simulink model "VCU10"  (R2021b)
settings: Solver=FixedStepDiscrete  StartTime=0.0  StopTime=10.0  FixedStep=0.01  RelTol=1e-3
values from neighbouring files (symbols this model uses):
  F = 0.0    [VCU10DB.sldd]
  FSEC_ESP_EMERGENCY_PRESSURE_MPA = 8.0    [VCU10DB.sldd]
  T = 1.0    [VCU10DB.sldd]
libraries: simulink x148, hdlsllib x90
(part 4 of 4)

== matlab function VCU10/DBC_Debug_StatusPack ==
  data: status_base input; status output; model_lox input; model_hox input
function status = dbg_status_pack(status_base, model_lox, model_hox)
%#codegen
status = uint8(status_base);
status(5) = uint8(model_lox);
status(6) = uint8(model_hox);
end

== stateflow chart VCU10/TS_Activation/Chart1 ==
  state Ignition_Check
    state begin
      run_flag=0;
    state Run_Check_Flag
      (default) -> (junction 5)
      (junction 5) -> (junction 7) [order 1] : [run_button==0]
      (junction 5) -> (junction 9) [order 2] : {run_check_flag=0;}
      (junction 7) -> (junction 8) : {run_check_flag=1;}
      (junction 8) -> (junction 9)
      (junction 9) -> (junction 10)
    state Check
      (default) -> (junction 23)
      (junction 23) -> (junction 25) [order 1] : [run_button==1]
      (junction 23) -> (junction 29) [order 2]
      (junction 25) -> (junction 27) : {run_flag=1;run=T;}
      (junction 27) -> (junction 29)
      (junction 29) -> (junction 32)
    (default) -> begin
    begin -> Run_Check_Flag
    (junction 17) -> Run_Check_Flag [order 2] : [run_check_flag==0]
    Check -> (junction 17)
    (junction 17) -> Check [order 1] : [run_check_flag==1]
    Run_Check_Flag -> (junction 17)
  state Flameout_Check
    state Run_Offcheck_Flag
      (default) -> (junction 39)
      (junction 39) -> (junction 42) [order 1] : [run_button==0]
      (junction 42) -> (junction 44) : {run_offcheck_flag=1;}
      (junction 39) -> (junction 46) [order 2] : {run_offcheck_flag}
      (junction 44) -> (junction 46)
      (junction 46) -> (junction 49)
    state Checkoff
      (default) -> (junction 63)
      (junction 63) -> (junction 61) [order 1] : [run_button==1]
      (junction 63) -> (junction 57) [order 2]
      (junction 61) -> (junction 60) : {run_flag=0;run=F;}
      (junction 60) -> (junction 57)
      (junction 57) -> (junction 58)
    (default) -> Run_Offcheck_Flag
    (junction 52) -> Run_Offcheck_Flag [order 1] : [run_offcheck_flag==0]
    (junction 52) -> Checkoff [order 3]
    (junction 52) -> Checkoff [order 2] : [run_offcheck_flag==1]
    Run_Offcheck_Flag -> (junction 52)
  (default) -> Ignition_Check
  Ignition_Check -> Flameout_Check : [run_flag==1]
  Flameout_Check -> Ignition_Check : [run_flag==0]
  data: run_button input; run output boolean; run_check_flag local =0; run_offcheck_flag local =0; run_flag local =0; T parameter; F parameter

== stateflow chart VCU10/TS_Activation/Chart2 ==
  state begin
  state delay
  (default) -> begin
  begin -> (junction 5) : {ts=0}
  (junction 5) -> (junction 11) : [tsms_button==1]
  (junction 11) -> (junction 35) : [di8==1]
  (junction 35) -> (junction 36) [order 2] : [as_flag==1]
  (junction 35) -> (junction 7) [order 1] : [as_flag==0]
  (junction 7) -> delay : [run==1&&brake_on==1]{ts=1;ts_warning=T}
  (junction 36) -> delay : {ts=1}
  delay -> (junction 30) : after(2,sec)
  (junction 30) -> (junction 9) : {ts_warning=F}
  (junction 9) -> (junction 13) : [tsms_button==0||di8==0||run==0]{ts=0}
  (junction 13) -> (junction 15)
  data: ts output; di8 input; run input; tsms_button input; brake_on input; ts_warning output; T parameter; F parameter; as_flag input

== stateflow chart VCU10/Res/Res_Msg/Subsystem/heaartbeat_chart ==
  state begin
  state compare
    res_hbcheck=1;
  state same
    hbcnt = hbcnt + 1;
  state judge
    res_hbcheck=0;
  (default) -> begin
  begin -> compare : [hasChanged(res_heartbeat)]
  judge -> compare : [hasChanged(res_heartbeat)]{hbcnt=0}
  same -> compare [order 2] : [hasChanged(res_heartbeat)]{hbcnt=0}
  compare -> same : [~hasChanged(res_heartbeat)]
  same -> judge [order 1] : [hbcnt>30]
  data: res_heartbeat input; res_hbcheck output; hbcnt local

== stateflow chart VCU10/Buzzer/Chart ==
  state Default
    en:
    ebs_buzzer=F;
  state Emergency
    en:
    ebs_buzzer=T;
  (default) -> Default
  Default -> Emergency : [as_emergency_flag==1]
  Emergency -> Default : [after(9,sec)]
  data: as_emergency_flag input; ebs_buzzer output; F parameter; T parameter

== matlab function VCU10/ASB_Selfcheck/FSEC_Sensor_Monitor ==
  data: brake_raw_mv input; brake_sensor_valid output; air_ready_raw_mv input; air_work_raw_mv input; air_ready_bar input; air_work_bar input; esp_ok input; res_ok input; ebs_driver_ok input; safety_fault output; brake_sensor_fault output; air_sensor_fault output; ebs_fault_indicator output
function [brake_sensor_valid, safety_fault, brake_sensor_fault, air_sensor_fault, ebs_fault_indicator] = fsec_sensor_monitor(brake_raw_mv, air_ready_raw_mv, air_work_raw_mv, air_ready_bar, air_work_bar, esp_ok, res_ok, ebs_driver_ok)
%#codegen
% 制动踏板为 0-5 V；两路气压为 0-10 V。阈值需在最终标定后复核。
persistent brake_bad brake_good air_bad air_good comm_bad comm_good ebs_bad ebs_good brake_fault air_fault comm_fault ebs_comm_fault
if isempty(brake_bad)
    brake_bad=uint16(0); brake_good=uint16(0); air_bad=uint16(0); air_good=uint16(0);
    comm_bad=uint16(0); comm_good=uint16(0); ebs_bad=uint16(0); ebs_good=uint16(0);
    brake_fault=false; air_fault=false; comm_fault=false; ebs_comm_fault=false;
end
brake_now = (brake_raw_mv < 100.0) || (brake_raw_mv > 4900.0);
if brake_now
    brake_good=uint16(0); if brake_bad<uint16(1000), brake_bad=brake_bad+uint16(1); end
    if brake_bad>=uint16(10), brake_fault=true; end
else
    brake_bad=uint16(0); if brake_good<uint16(1000), brake_good=brake_good+uint16(1); end
    if brake_good>=uint16(50), brake_fault=false; end
end
% 储气侧低压可直接阻止 Ready；下游低压仅在 EBS 触发后由响应监控判断。
air_now = (air_ready_raw_mv > 9800.0) || (air_work_raw_mv > 9800.0) || ...
          (air_ready_bar < 2.5) || (air_work_bar > air_ready_bar + 1.5);
if air_now
    air_good=uint16(0); if air_bad<uint16(1000), air_bad=air_bad+uint16(1); end
    if air_bad>=uint16(50), air_fault=true; end
else
    air_bad=uint16(0); if air_good<uint16(1000), air_good=air_good+uint16(1); end
    if air_good>=uint16(50), air_fault=false; end
end
comm_now = (~logical(esp_ok)) || (~logical(res_ok)) || (~logical(ebs_driver_ok));
if comm_now
    comm_good=uint16(0); if comm_bad<uint16(1000), comm_bad=comm_bad+uint16(1); end
    if comm_bad>=uint16(30), comm_fault=true; end
else
    comm_bad=uint16(0); if comm_good<uint16(1000), comm_good=comm_good+uint16(1); end
    if comm_good>=uint16(50), comm_fault=false; end
end
% EBS 红灯只显示 EBS/制动冗余本体故障，不显示 RES 一般安全事件。
ebs_comm_now = (~logical(esp_ok)) || (~logical(ebs_driver_ok));
if ebs_comm_now
    ebs_good=uint16(0); if ebs_bad<uint16(1000), ebs_bad=ebs_bad+uint16(1); end
    if ebs_bad>=uint16(30), ebs_comm_fault=true; end
else
    ebs_bad=uint16(0); if ebs_good<uint16(1000), ebs_good=ebs_good+uint16(1); end
    if ebs_good>=uint16(50), ebs_comm_fault=false; end
end
brake_sensor_valid = (~brake_fault) && (~brake_now);
brake_sensor_fault = brake_fault;
air_sensor_fault = air_fault;
safety_fault = brake_fault || air_fault || comm_fault;
ebs_fault_indicator = brake_fault || air_fault || ebs_comm_fault;
end

== stateflow chart VCU10/LED_Control/Subsystem/blue ==
  state Delay
    en:
    blue=uint16(60000);
  state Node
    en:
    blue=uint16(0);
  state Close
    en:
    blue=uint16(0);
  state On
    en:
    blue=uint16(60000);
  state Blink
    en:
    blue=uint16(30000);
  (default) -> Delay
  Delay -> Node : after(2,sec)
  Node -> Close [order 2] : [as_led_blue==0]
  Node -> Blink [order 3] : [as_led_blue==2]
  Node -> On [order 1] : [as_led_blue==1]
  Close -> On [order 1] : [as_led_blue==1]
  On -> Blink [order 1] : [as_led_blue==2]
  Blink -> On [order 2] : [as_led_blue==1]
  On -> Close [order 2] : [as_led_blue==0]
  Close -> Blink [order 2] : [as_led_blue==2]
  Blink -> Close [order 1] : [as_led_blue==0]
  data: as_led_blue input; blue output; asms_button input

== stateflow chart VCU10/LED_Control/Subsystem1/yellow ==
  state delay
    en:
    yellow=uint16(60000);
  state node
    en:
    yellow=uint16(0);
  state Close
    en:
    yellow=uint16(0);
  state On
    en:
    yellow=uint16(60000);
  state Blink
    en:
    yellow=uint16(30000);
  (default) -> delay
  delay -> node : after(2,sec)
  node -> Blink [order 3] : [as_led_yellow==2]
  node -> Close [order 2] : [as_led_yellow==0]
  node -> On [order 1] : [as_led_yellow==1]
  Close -> On [order 1] : [as_led_yellow==1]
  On -> Blink [order 1] : [as_led_yellow==2]
  Blink -> On [order 2] : [as_led_yellow==1]
  On -> Close [order 2] : [as_led_yellow==0]
  Close -> Blink [order 2] : [as_led_yellow==2]
  Blink -> Close [order 1] : [as_led_yellow==0]
  data: as_led_yellow input; yellow output; asms_button input

== stateflow chart VCU10/EPS/EPS_TransmitMsg/EPS_Stateflow1 ==
  state EPS_Unable
    en:
    eps_cmdworkmode=0x00;
    eps_cmdmiddle=0x00;
  state EPS_Enable
    en:
    eps_cmdworkmode=0x10;
    eps_cmdangle=ipc_cmdangle;
    eps_cmdmiddle=0x00;
    eps_cmdvelocity=ipc_eps_velocity;
    du:
    eps_cmdworkmode=0x10;
    eps_cmdangle=ipc_cmdangle;
    eps_cmdmiddle=0x00;
    eps_cmdvelocity=ipc_eps_velocity;
  state EPS_Return
    eps_cmdworkmode=0x10;
    eps_cmdangle=uint32(0x04);
    eps_cmdmiddle=0x55;
    eps_cmdvelocity=0x14;
  (default) -> EPS_Unable
  EPS_Enable -> EPS_Unable [order 1] : [steering_flag==0]
  EPS_Unable -> EPS_Enable : [steering_flag==1]
  EPS_Enable -> (junction 22) [order 2] : [after(10,msec)]
  (junction 22) -> EPS_Return : [steer_return==1]
  EPS_Return -> EPS_Enable : [steer_zero==1]
  data: eps_cmdworkmode output; steering_flag input; steer_return input; ipc_cmdangle input; ipc_eps_velocity input; steer_zero input; eps_cmdangle output; eps_cmdmiddle output; eps_cmdvelocity output

== stateflow chart VCU10/ESP/ESP_TransmitMsg/ESP_R_00/ESP_Chart1 ==
  state ESC_Unable
    en:
    mode=0;
    %mode=机械模式;
  state ESC_Engage
    en:
    %开环模式;
    mode=1;
    tarPrsReqFL=ipc_esp_flprs;
    tarPrsReqFR=ipc_esp_frprs;
    tarPrsReqRL=ipc_esp_rlprs;
    tarPrsReqRR=ipc_esp_rrprs;
    du:
    mode=1;
    tarPrsReqFL=ipc_esp_flprs;
    tarPrsReqFR=ipc_esp_frprs;
    tarPrsReqRL=ipc_esp_rlprs;
    tarPrsReqRR=ipc_esp_rrprs;
  state ESC_Able
    en:
    %开环模式;
    mode=1;
    tarPrsReqFL=ipc_esp_flprs;
    tarPrsReqFR=ipc_esp_frprs;
    tarPrsReqRL=ipc_esp_rlprs;
    tarPrsReqRR=ipc_esp_rrprs;
    du:
    mode=1;
    tarPrsReqFL=ipc_esp_flprs;
    tarPrsReqFR=ipc_esp_frprs;
    tarPrsReqRL=ipc_esp_rlprs;
    tarPrsReqRR=ipc_esp_rrprs;
  (default) -> ESC_Unable
  ESC_Able -> ESC_Unable : [brake_flag==0]
  ESC_Unable -> ESC_Engage : [brake_flag==2]
  ESC_Engage -> ESC_Able : [brake_flag==1]
  data: ipc_esp_flprs input; ipc_esp_frprs input; ipc_esp_rlprs input; ipc_esp_rrprs input; brake_flag input; tarPrsReqFL output; tarPrsReqFR output; tarPrsReqRL output; tarPrsReqRR output; mode output

== stateflow chart VCU10/LED_Control/EBS_LED/Shutdown_Button ==
  state begin
  state same1
    shutdown_flag=T;
  state compare
    shutdown_count = shutdown_count + 1;
  state judge
    shutdown_flag=F;
  (default) -> begin
  begin -> (junction 28) : after(1,sec)
  (junction 28) -> same1 : [Shutdown_Start==Shutdown_End]
  judge -> same1 : [Shutdown_Start==Shutdown_End]
  compare -> same1 [order 2] : [Shutdown_Start==Shutdown_End]{shutdown_count=0}
  same1 -> compare : [Shutdown_Start~=Shutdown_End]
  compare -> judge [order 1] : [shutdown_count>10]
  data: Shutdown_Start input; shutdown_flag output; Shutdown_End input; shutdown_count local =0; F parameter; T parameter

== stateflow chart VCU10/ESP/ESP_ReceiveMsg/Subsystem/brkmotor_check_system ==
  state begin
  state compare
    brkmotor_check=T;
  state same
    lscnt = lscnt + 1;
  state judge
    brkmotor_check=F;
  (default) -> begin
  begin -> compare : [hasChanged(lifesig)]
  judge -> compare : [hasChanged(lifesig)]{lscnt=0}
  same -> compare [order 2] : [hasChanged(lifesig)]{lscnt=0}
  compare -> same : [~hasChanged(lifesig)]
  same -> judge [order 1] : [lscnt>10]
  data: lifesig input; brkmotor_check output; lscnt local; T parameter; F parameter

== stateflow chart VCU10/Res/Res_Msg/Subsystem/xor_Check ==
  state compare
    en:
    xorcheck=1;
  state Init
    en:
    err_cnt=0;
  state different
    en:
    err_cnt = err_cnt + 1;
  state judge
    en:
    xorcheck=0;
  (default) -> Init
  Init -> compare : [res_xorcheck==xor_consequence]
  judge -> compare : [res_xorcheck==xor_consequence]{err_cnt=0}
  compare -> different : [res_xorcheck~=xor_consequence]
  different -> compare [order 2] : [res_xorcheck==xor_consequence]{err_cnt=0}
  different -> judge [order 1] : [err_cnt>=10]
  data: res_xorcheck input; xor_consequence input; xorcheck output; err_cnt local

== stateflow chart VCU10/AMI_CAN/AMI_Transmitmsg/Chart ==
  state as_off
    en:
    ami_process=0x01
  state as_emergency
    en:
    ami_process=0x40
  state begin
  state munual_driving
    en:
    ami_process=0x02
  state as_finished
    en:
    ami_process=0x20
  state as_ready
    en:
    ami_process=0x04
  state as_driving
    en:
    ami_process=0x10
  state r2d
    en:
    ami_process=0x08
  begin -> as_off [order 1] : [as_off_flag==1]
  begin -> as_emergency [order 7] : [as_emergency_flag==1]
  as_emergency -> begin : [as_emergency_flag~=1]
  as_off -> begin : [as_off_flag~=1]
  (default) -> begin
  begin -> munual_driving [order 2] : [munual_driving_flag==1]
  begin -> as_finished [order 6] : [as_finished_flag==1]
  munual_driving -> begin : [munual_driving_flag~=1]
  as_finished -> begin : [as_finished_flag~=1]
  begin -> as_ready [order 3] : [as_ready_flag==1]
  as_ready -> begin : [as_ready_flag~=1]
  begin -> r2d [order 4] : [r2d_flag==1]
  r2d -> begin : [r2d_flag~=1]
  begin -> as_driving [order 5] : [as_driving_flag==1]
  as_driving -> begin : [as_driving_flag~=1]
  data: as_off_flag input; munual_driving_flag input; as_ready_flag input; r2d_flag input; as_driving_flag input; as_finished_flag input; as_emergency_flag input; ami_process output

== stateflow chart VCU10/Motor_Control/ManualTorque_Calculation/Pedal_Fault_Check ==
  (default) -> (junction 1)
  (junction 1) -> (junction 5) [order 1] : [abs(apps1-apps2)>=0.1]{fault_count = fault_count + 1}
  (junction 5) -> (junction 3) [order 2]
  (junction 1) -> (junction 3) [order 2] : {fault_count=0;pedal_error=0}
  (junction 5) -> (junction 10) [order 1] : [fault_count>=10]{pedal_error=1}
  (junction 10) -> (junction 3)
  (junction 3) -> (junction 13)
  data: apps1 input; apps2 input; pedal_error output; fault_count local =0

== matlab function VCU10/EBS/EBS_Response_Monitor ==
  data: trigger input; ebs_sensor_fault output; asms input; driver_ok input; air_ready_bar input; air_work_bar input
function ebs_sensor_fault = ebs_response_monitor(trigger, asms, driver_ok, air_ready_bar, air_work_bar)
%#codegen
% EBS_Driver 负责电气诊断；VCU 校验触发后的气动建压响应。
persistent last_trigger waiting wait_count relation_count clear_count fault_latched
if isempty(last_trigger)
    last_trigger=false; waiting=false; wait_count=uint16(0); relation_count=uint16(0);
    clear_count=uint16(0); fault_latched=false;
end
rising = logical(trigger) && ~last_trigger; last_trigger=logical(trigger);
if rising && logical(driver_ok) && (air_ready_bar >= 2.5) && (air_work_bar < 1.0)
    waiting=true; wait_count=uint16(0);
end
if waiting
    if air_work_bar >= 1.0
        waiting=false; wait_count=uint16(0);
    else
        if wait_count<uint16(1000), wait_count=wait_count+uint16(1); end
        if wait_count>=uint16(20), fault_latched=true; waiting=false; end
    end
end
if air_work_bar > air_ready_bar + 1.5
    if relation_count<uint16(1000), relation_count=relation_count+uint16(1); end
    if relation_count>=uint16(20), fault_latched=true; end
else
    relation_count=uint16(0);
end
if (~logical(asms)) && logical(driver_ok) && (air_work_bar < 1.0) && (air_ready_bar >= 2.5)
    if clear_count<uint16(1000), clear_count=clear_count+uint16(1); end
    if clear_count>=uint16(100), fault_latched=false; end
else
    clear_count=uint16(0);
end
ebs_sensor_fault = fault_latched;
end

== matlab function VCU10/EPS_SCS_Monitor ==
  data: msg1 input; eps_safety_fault output; msg2 input
function eps_safety_fault = eps_scs_monitor(msg1, msg2)
%#codegen
% 0x401: Byte7 = XOR(Byte0..Byte6); 0x402: Byte1 为发送计数。
persistent last_counter seen_count stale_count bad_count good_count fault
if isempty(last_counter)
    last_counter=msg2(2); seen_count=uint16(0); stale_count=uint16(0);
    bad_count=uint16(0); good_count=uint16(0); fault=true;
end
counter=msg2(2);
if counter~=last_counter
    last_counter=counter; stale_count=uint16(0);
    if seen_count<uint16(1000), seen_count=seen_count+uint16(1); end
else
    if stale_count<uint16(1000), stale_count=stale_count+uint16(1); end
end
checksum=uint8(0);
for k=1:7
    checksum=bitxor(checksum,msg1(k));
end
content_valid=(checksum==msg1(8)) && (msg1(3)==uint8(0)) && (msg1(7)==uint8(0));
fresh=(seen_count>=uint16(3)) && (stale_count<uint16(30));
valid_now=content_valid && fresh;
if valid_now
    bad_count=uint16(0); if good_count<uint16(1000), good_count=good_count+uint16(1); end
    if good_count>=uint16(50), fault=false; end
else
    good_count=uint16(0); if bad_count<uint16(1000), bad_count=bad_count+uint16(1); end
    if (bad_count>=uint16(3)) || (stale_count>=uint16(30)), fault=true; end
end
eps_safety_fault=fault;
end

== matlab function VCU10/Motor_Control/ManualTorque_Calculation/APPS_Electrical_Monitor ==
  data: apps1_raw_mv input; apps_valid output; apps2_raw_mv input; apps_electrical_fault output
function [apps_valid, apps_electrical_fault] = apps_electrical_monitor(apps1_raw_mv, apps2_raw_mv)
%#codegen
% 0-5 V APPS 单通道开路/短路诊断；最终阈值由实车标定确认。
persistent bad_count good_count fault
if isempty(bad_count)
    bad_count=uint16(0); good_count=uint16(0); fault=false;
end
bad_now=(apps1_raw_mv<100.0)||(apps1_raw_mv>4900.0)||...
        (apps2_raw_mv<100.0)||(apps2_raw_mv>4900.0);
if bad_now
    good_count=uint16(0); if bad_count<uint16(1000), bad_count=bad_count+uint16(1); end
    if bad_count>=uint16(10), fault=true; end
else
    bad_count=uint16(0); if good_count<uint16(1000), good_count=good_count+uint16(1); end
    if good_count>=uint16(50), fault=false; end
end
apps_valid=(~bad_now) && (~fault);
apps_electrical_fault=fault;
end
